simulink model "RLC_system"  (R2020a)
settings: Solver=VariableStepAuto  StartTime=0.0  StopTime=10.0  RelTol=1e-3
settings Model: Creator=User  LastModifiedBy=User

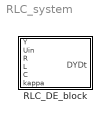
== system RLC_system ==
  RLC_DE_block : MATLAB Function  TreatAsAtomicUnit=on

== matlab function RLC_system/RLC_DE_block ==
  data: Y input; DYDt output; Uin input; R input; L input; C input; kappa input
function DYDt = RLC_DE_block(Y,Uin,R,L,C,kappa)
%#codegen

%    This function was generated by the Symbolic Math Toolbox version 8.5.
%    12-Dec-2020 10:36:27

t2 = Y(1);
t3 = Y(2);
DYDt = [t3;-(-Uin+t2+kappa.*t2.^3+C.*R.*t3)./(C.*L)];
